simulink model "Control_System_2016a"  (R2016a)
settings: Solver=VariableStepAuto  StartTime=0.0  StopTime=10.0  RelTol=1e-3
libraries: simulink x1
settings Model: Creator=univ4123  LastModifiedBy=univ4123

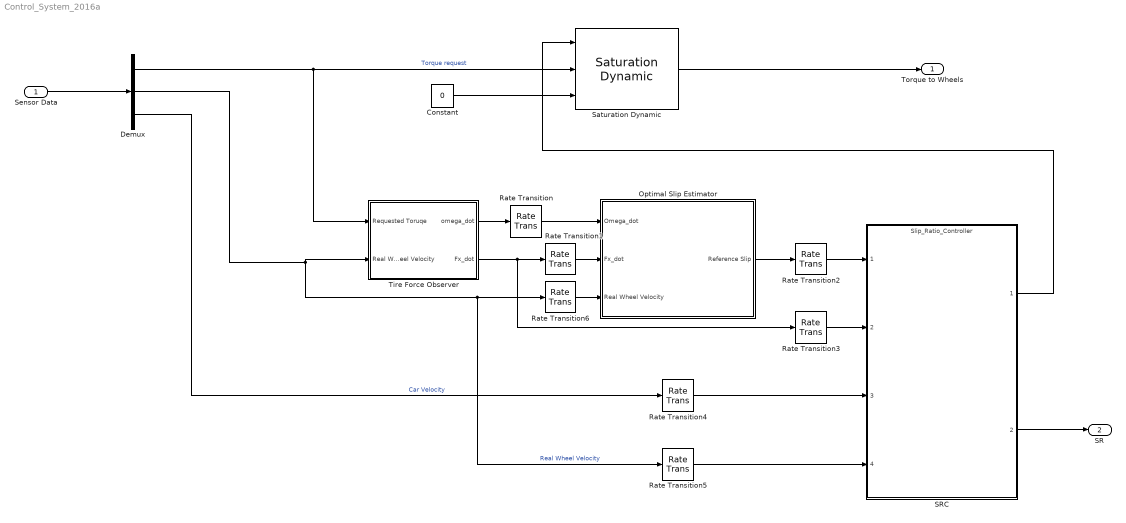
== system Control_System_2016a ==
  Sensor Data : Inport
  Constant : Constant  Value=0
  Demux : Demux  Outputs=3
  Optimal Slip Estimator : Subsystem
  Rate Transition : RateTransition  OutPortSampleTime=OSE_Ts
  Rate Transition1 : RateTransition  OutPortSampleTime=OSE_Ts
  Rate Transition{2..5} (4 alike) : RateTransition  OutPortSampleTimeOpt=Inherit
  Rate Transition6 : RateTransition  OutPortSampleTime=OSE_Ts
  SRC : ModelReference  ModelNameDialog=Slip_Ratio_Controller.slx  SimulationMode=Normal  ModelReferenceVersion=1.1
  Saturation Dynamic : simulink/Discontinuities/Saturation Dynamic  OutMin=[]  OutMax=[]  OutDataTypeStr=Inherit: Same as second input  OutDataType=fixdt(1, 16)  OutScaling=2^-10  DoSatur=off
  Tire Force Observer : Subsystem
  Torque to Wheels : Outport
  SR : Outport  Port=2
  wires:
  Demux/1 -> Tire Force Observer/1(Requested Toruqe), Saturation Dynamic/2  "Torque request"
  Saturation Dynamic/1 -> Torque to Wheels/1
  Tire Force Observer/1(omega_dot) -> Rate Transition/1
  SRC/1 -> Saturation Dynamic/1
  Constant/1 -> Saturation Dynamic/3
  Tire Force Observer/2(Fx_dot) -> Rate Transition3/1, Rate Transition1/1
  Sensor Data/1 -> Demux/1
  Demux/2 -> Tire Force Observer/2(Real Wheel Velocity), Rate Transition6/1, Rate Transition5/1  "Real Wheel Velocity"
  Optimal Slip Estimator/1(Reference Slip) -> Rate Transition2/1
  Demux/3 -> Rate Transition4/1  "Car Velocity"
  SRC/2 -> SR/1
  Rate Transition/1 -> Optimal Slip Estimator/1(Omega_dot)
  Rate Transition1/1 -> Optimal Slip Estimator/2(Fx_dot)
  Rate Transition2/1 -> SRC/1
  Rate Transition3/1 -> SRC/2
  Rate Transition4/1 -> SRC/3
  Rate Transition5/1 -> SRC/4
  Rate Transition6/1 -> Optimal Slip Estimator/3(Real Wheel Velocity)

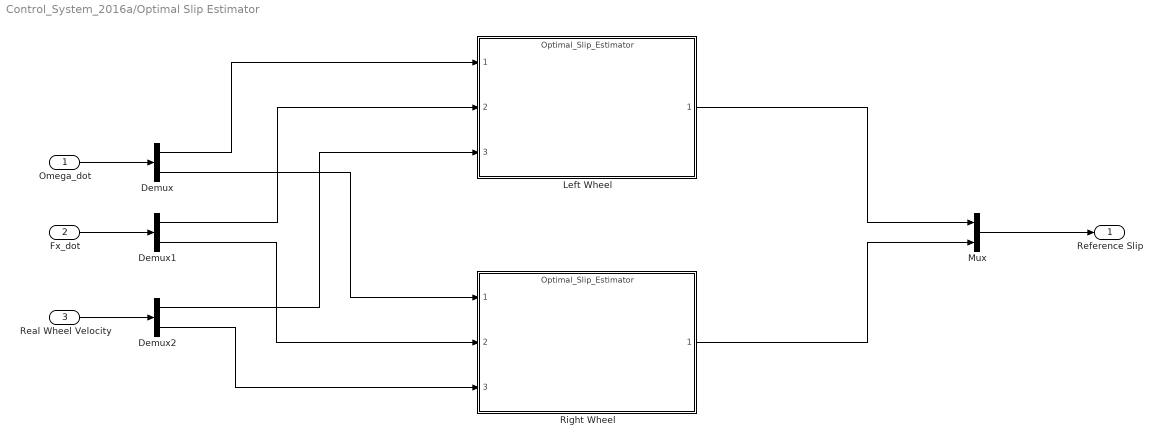
== system Control_System_2016a/Optimal Slip Estimator ==
  Omega_dot : Inport
  Fx_dot : Inport  Port=2
  Real Wheel Velocity : Inport  Port=3
  Demux : Demux  Outputs=2
  Demux1 : Demux  Outputs=2
  Demux2 : Demux  Outputs=2
  Left Wheel : ModelReference  ModelNameDialog=Optimal_Slip_Estimator  SimulationMode=Normal  ModelReferenceVersion=1.4
  Mux : Mux  Inputs=2
  Right Wheel : ModelReference  ModelNameDialog=Optimal_Slip_Estimator  SimulationMode=Normal  ModelReferenceVersion=1.4
  Reference Slip : Outport
  wires:
  Mux/1 -> Reference Slip/1
  Omega_dot/1 -> Demux/1
  Demux/1 -> Left Wheel/1
  Demux/2 -> Right Wheel/1
  Fx_dot/1 -> Demux1/1
  Real Wheel Velocity/1 -> Demux2/1
  Demux2/1 -> Left Wheel/3
  Demux2/2 -> Right Wheel/3
  Demux1/1 -> Left Wheel/2
  Demux1/2 -> Right Wheel/2
  Left Wheel/1 -> Mux/1
  Right Wheel/1 -> Mux/2

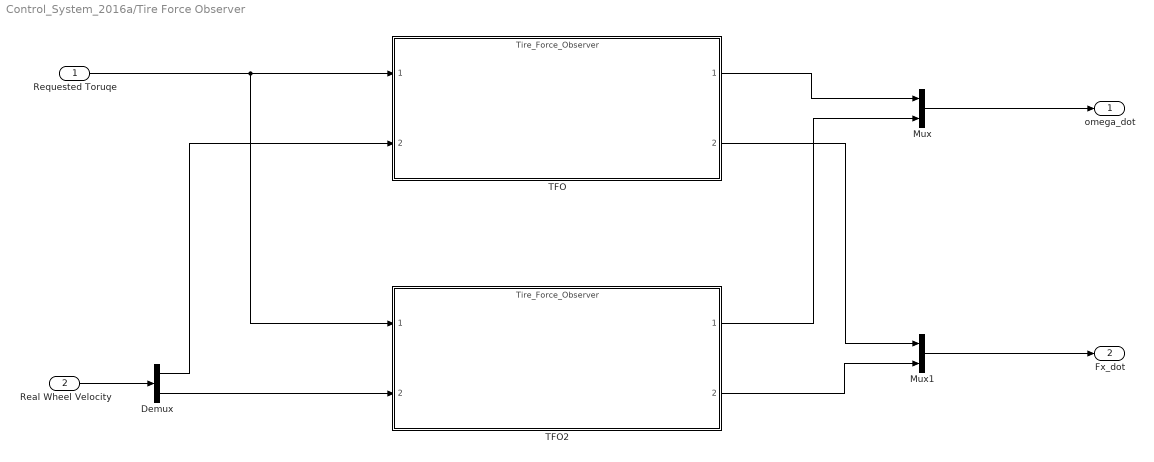
== system Control_System_2016a/Tire Force Observer ==
  Requested Toruqe : Inport
  Real Wheel Velocity : Inport  Port=2
  Demux : Demux  Outputs=2
  Mux : Mux  Inputs=2
  Mux1 : Mux  Inputs=2
  TFO : ModelReference  ModelNameDialog=Tire_Force_Observer.slx  SimulationMode=Normal  ModelReferenceVersion=1.3
  TFO2 : ModelReference  ModelNameDialog=Tire_Force_Observer.slx  SimulationMode=Normal  ModelReferenceVersion=1.3
  omega_dot : Outport
  Fx_dot : Outport  Port=2
  wires:
  Requested Toruqe/1 -> TFO2/1, TFO/1
  Real Wheel Velocity/1 -> Demux/1
  Demux/1 -> TFO/2
  Demux/2 -> TFO2/2
  TFO2/1 -> Mux/2
  TFO/1 -> Mux/1
  TFO/2 -> Mux1/1
  TFO2/2 -> Mux1/2
  Mux/1 -> omega_dot/1
  Mux1/1 -> Fx_dot/1
